simulink model "A14_Servoachse_PID"  (R2017b)
settings: Solver=ode45  StartTime=0.0  StopTime=10  FixedStep=0.001  MaxStep=1e-4  RelTol=1e-3  EnableMultiTasking=on
values from neighbouring files (symbols this model uses):
  CD = 1e1    (= 10)    [A14_Konstanten.m]    (also in A17_Konstanten.m = 100; A8_Konstanten.m = 20; A9_Konstanten.m = 0.1)
  CF = 1e4    (= 10000)    [A13_Konstanten.m]    (also in A14_Konstanten.m; A17_Konstanten.m = 50000; A8_Konstanten.m = 10000000; A9_Konstanten.m)
  CM = 7.1e-7    (= 7.1e-07)    [A10_Konstanten.m]    (also in A13_Konstanten.m; A14_Konstanten.m; A16_Konstanten.m)
  CR = 0.2    [A13_Konstanten.m]    (also in A14_Konstanten.m; A17_Konstanten.m = 100; A9_Konstanten.m = 1; Z_Parametrisierung_Skript.m = [0.5,1,5])
  FReib = 0.5    [A13_Konstanten.m]    (also in A14_Konstanten.m)
  Imax = 4.81    [A10_Konstanten.m]    (also in A13_Konstanten.m; A14_Konstanten.m; A16_Konstanten.m)
  JM = JR + JG    (= 1.38e-06)    [A13_Konstanten.m]    (also in A14_Konstanten.m)
  KM = 38.4e-3    (= 0.0384)    [A10_Konstanten.m]    (also in A13_Konstanten.m; A14_Konstanten.m; A16_Konstanten.m)
  KN = 1/(2*pi*KM)    (= 4.14465997635)    [A10_Konstanten.m]    (also in A13_Konstanten.m; A14_Konstanten.m; A16_Konstanten.m)
  LA = 4.64e-4    (= 0.000464)    [A10_Konstanten.m]    (also in A13_Konstanten.m; A14_Konstanten.m; A16_Konstanten.m)
  m1 = 1    [A13_Konstanten.m]    (also in A14_Konstanten.m; A17_Konstanten.m = 4; A8_Konstanten.m = 20)
  R = 0.02    [A10_Konstanten.m]    (also in A13_Konstanten.m = 0.04; A14_Konstanten.m = 0.04; A16_Konstanten.m)
  RA = 4.99    [A10_Konstanten.m]    (also in A13_Konstanten.m; A14_Konstanten.m; A16_Konstanten.m)
  TPWM = 2e-5    (= 2e-05)    [A14_Konstanten.m]
  Tssens = Tnsens    (= 8e-05)    [A14_Konstanten.m]
  Ue = 4    [A13_Konstanten.m]    (also in A14_Konstanten.m)
  Umax = 24    [A10_Konstanten.m]    (also in A13_Konstanten.m; A14_Konstanten.m; A16_Konstanten.m; A17_Konstanten.m = 120)
  WGrad = 0.85    [A13_Konstanten.m]    (also in A14_Konstanten.m)
undefined symbols (not defined in the file or in its folder): sigbuilder_block
libraries: simulink x2
settings Model: Creator=jbaur  LastModifiedBy=jbaur
settings DataIOCC: ExternalInput=X1  SaveFormat=StructureWithTime  InspectSignalLogs=on  SignalLoggingName=sigsOut
settings OptimizationCC: DefaultParameterBehavior=Inlined  InlineInvariantSignals=on  BufferReuse=off  ExpressionDepthLimit=2147483647  InitFltsAndDblsToZero=on  LifeSpan=inf
settings DebuggingCC: SaveWithParameterizedLinksMsg=none  SignalResolutionControl=TryResolveAllWithWarning  MultiTaskDSMMsg=warning  MultiTaskCondExecSysMsg=none  StateNameClashWarn=warning  InitInArrayFormatMsg=none  SFUnexpectedBacktrackingDiag=warning  SFNoUnconditionalDefaultTransitionDiag=warning  SFExecutionAtInitializationDiag=none
settings HardwareCC: ProdBitPerPointer=32  ProdBitPerSizeT=32  ProdBitPerPtrDiffT=32  ProdLargestAtomicFloat=None  ProdIntDivRoundTo=Undefined  ProdEndianess=Unspecified  ProdWordSize=32  ProdHWDeviceType=32-bit Generic  TargetUnknown=on
settings ModelReferenceCC: PropagateSignalLabelsOutOfModel=off
settings CodeAppCC: StateflowObjectComments=on
settings GRTTargetCC: TargetFcnLib=ansi_tfl_tmw.mat  TargetLangStandard=C89/C90 (ANSI)  ModelReferenceCompliant=off  GeneratePreprocessorConditionals=Disable all  CombineOutputUpdateFcns=off  MatFileLogging=off  GRTInterface=on
settings ConfigComp: CovMetricSettings=dw  CovHtmlReporting=on  CovSaveCumulativeToWorkspaceVar=on  CovSaveSingleToWorkspaceVar=on  CovExternalEMLEnable=off  CovSFcnEnable=off

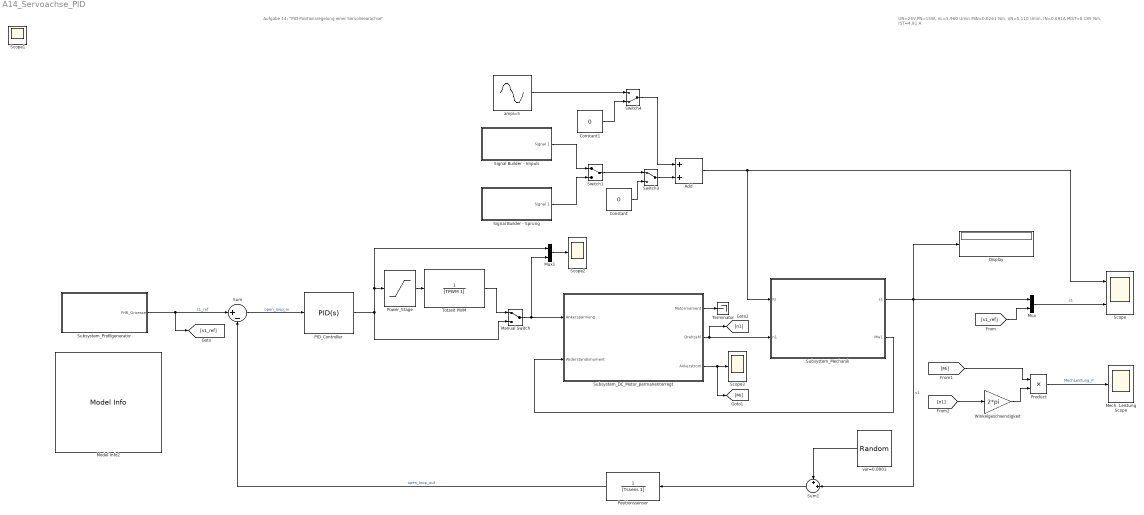
== system A14_Servoachse_PID ==
  note: Aufgabe 14: "PID-Positionsregelung einer Servolinearachse"
  note: UN=24V,PN=15W, nL=5.960 Umin
      | MiN=0.0261 Nm, nN=5.110 Umin, IN=0.691A
      | MiST=0.185 Nm, IST=4.81 A
  Add : Sum
  Constant : Constant  Value=0
  Constant1 : Constant  Value=0
  Display : Display
  Manual Switch : ManualSwitch
  Mech. Leistung Scope : Scope
  Model Info2 : simulink/Model-Wide Utilities/Model Info  Frame=on  DisplayStringWithTags=|  HorizontalTextAlignment=Left  LeftAlignmentValue=0.02
      | Bewegungsprofil:
      | ------------------------
      | Tmax = 1s
      | smax = 0,5m
      | vmax = 1 m/s
      | amax = 2 m/s^2
  Mux : Mux  Inputs=2
  Mux1 : Mux  Inputs=2
  PID_Controller : simulink/Continuous/PID Controller  Controller=PID  TimeDomain=Continuous-time  SampleTime=-1  IntegratorMethod=Forward Euler  FilterMethod=Forward Euler  Form=Ideal  UseFilter=on  ControllerParametersSource=internal  P=10  I=1  D=0  N=1000  InitialConditionSource=internal  InitialConditionForIntegrator=0  InitialConditionForFilter=0  ExternalReset=none  LimitOutput=off  UpperSaturationLimit=Umax  LowerSaturationLimit=-Umax  LinearizeAsGain=off  AntiWindupMode=clamping  Kb=1  TrackingMode=off  Kt=1  PParamMin=[]  PParamMax=[]  IParamMin=[]  IParamMax=[]  DParamMin=[]  DParamMax=[]  NParamMin=[]  NParamMax=[]  KbParamMin=[]  KbParamMax=[]  KtParamMin=[]  KtParamMax=[]  POutMin=[]  POutMax=[]  IOutMin=[]  IOutMax=[]  DOutMin=[]  DOutMax=[]  NOutMin=[]  NOutMax=[]  KbOutMin=[]  KbOutMax=[]  KtOutMin=[]  KtOutMax=[]  IntegratorOutMin=[]  IntegratorOutMax=[]  FilterOutMin=[]  FilterOutMax=[]  SumOutMin=[]  SumOutMax=[]  SumI1OutMin=[]  SumI1OutMax=[]  SumI2OutMin=[]  SumI2OutMax=[]  SumI3OutMin=[]  SumI3OutMax=[]  SumDOutMin=[]  SumDOutMax=[]  SaturationOutMin=[]  SaturationOutMax=[]  IntegratorContinuousStateAttributes=''  IntegratorStateMustResolveToSignalObject=off  IntegratorRTWStateStorageClass=Auto  FilterContinuousStateAttributes=''  FilterStateMustResolveToSignalObject=off  FilterRTWStateStorageClass=Auto  DifferentiatorICPrevScaledInput=0  DifferentiatorOutMin=[]  DifferentiatorOutMax=[]  InitialConditionSetting=State (most efficient)  FilterDiffOutCoefMin=[]  FilterDiffOutCoefMax=[]  SumDenOutMin=[]  SumDenOutMax=[]  SumNumOutMin=[]  SumNumOutMax=[]  ReciprocalOutMin=[]  ReciprocalOutMax=[]  DivideOutMin=[]  DivideOutMax=[]  TunerSelectOption=Transfer Function Based (PID Tuner App)
  Positionssensor : TransferFcn  Denominator=[Tssens 1]
  Power_Stage : Saturate  UpperLimit=Umax  LowerLimit=-Umax
  Product : Product  RndMeth=Zero
  Scope : Scope  NumInputPorts=2
  Scope2 : Scope
  Scope3 : Scope
  Signal Builder - Impuls : Subsystem  Tag=STV Subsys  LoadFcn=sigbuilder_block('load');  StartFcn=sigbuilder_block('start');  StopFcn=sigbuilder_block('stop');  ClipboardFcn=sigbuilder_block('clipboard');  mask(Sigbuilder block){tuvar=[0:10]}
      mask help: Simulink:masks:SigbuilderBlock_MD
      mask init:
      | if ~strcmp(get_param(bdroot(gcbh),'SimulationStatus'),'stopped') tuvar = sigbuilder_block('maskInit'); end
      settings: CopyFcn=sigbuilder_block('copy');  DeleteFcn=sigbuilder_block('delete');  ModelCloseFcn=sigbuilder_block('modelClose');  PreSaveFcn=sigbuilder_block('preSave');  PauseFcn=sigbuilder_block('pause');  ContinueFcn=sigbuilder_block('continue');  NameChangeFcn=sigbuilder_block('namechange');  OpenFcn=sigbuilder_block('open',[431.25 106.5 550.5 399.75 ]);  CloseFcn=sigbuilder_block('close');
      mask Display: plot(0, 0, 100, 100,[2, 2, 32, 32, 2], [68, 8, 8, 68, 68],[32, 2], [38, 38], [32, 19, 2],[53, 60, 44], [32, 17, 17, 2],[16, 16, 31, 31]);txt = getActiveGroup(gcbh);text(2, 100, txt,'verticalAlignment', 'top');
  Signal Builder - Sprung : Subsystem  Tag=STV Subsys  LoadFcn=sigbuilder_block('load');  StartFcn=sigbuilder_block('start');  StopFcn=sigbuilder_block('stop');  ClipboardFcn=sigbuilder_block('clipboard');  mask(Sigbuilder block){tuvar=[0:10]}
      mask help: Simulink:masks:SigbuilderBlock_MD
      mask init:
      | if ~strcmp(get_param(bdroot(gcbh),'SimulationStatus'),'stopped') tuvar = sigbuilder_block('maskInit'); end
      settings: CopyFcn=sigbuilder_block('copy');  DeleteFcn=sigbuilder_block('delete');  ModelCloseFcn=sigbuilder_block('modelClose');  PreSaveFcn=sigbuilder_block('preSave');  PauseFcn=sigbuilder_block('pause');  ContinueFcn=sigbuilder_block('continue');  NameChangeFcn=sigbuilder_block('namechange');  OpenFcn=sigbuilder_block('open',[1699.5 180.75 550.5 399.75 ]);  CloseFcn=sigbuilder_block('close');
      mask Display: plot(0, 0, 100, 100,[2, 2, 32, 32, 2], [68, 8, 8, 68, 68],[32, 2], [38, 38], [32, 19, 2],[53, 60, 44], [32, 17, 17, 2],[16, 16, 31, 31]);txt = getActiveGroup(gcbh);text(2, 100, txt,'verticalAlignment', 'top');
  Subsystem_DC_Motor_permanenterregt : Subsystem
  Subsystem_Mechanik : Subsystem
  Subsystem_Profilgenerator : Subsystem
  Sum : Sum  Inputs=|+-  SaturateOnIntegerOverflow=on
  Sum1 : Sum  Inputs=++|
  Switch1 : ManualSwitch
  Switch3 : ManualSwitch
  Switch4 : ManualSwitch  CurrentSetting=0
  Terminator : Terminator
  Totzeit PWM : TransferFcn  Denominator=[TPWM 1]
  Winkelgeschwindigkeit : Gain  Gain=2*pi
  ampl=5 : Sin  Amplitude=5  Frequency=2*pi*20  SampleTime=0
  var=0.0001 : RandomNumber  Variance=0  SampleTime=0.001
  Scope1 : Scope
  wires:
  Sum/1 -> PID_Controller/1  "open_loop_in"
  Subsystem_Profilgenerator/1(FHR_Groesse) -> Sum/1, [s1_ref]  "s1_ref"
  Mux/1 -> Scope/2  "s1"
  Power_Stage/1 -> Totzeit PWM/1
  Manual Switch/1 -> Subsystem_DC_Motor_permanenterregt/1(Ankerspannung), Mux1/2
  Subsystem_DC_Motor_permanenterregt/2(Drehzahl) -> Subsystem_Mechanik/2(n1), [n1]
  Subsystem_Mechanik/2(Mw1) -> Subsystem_DC_Motor_permanenterregt/2(Widerstandsmoment)
  Mux1/1 -> Scope2/1
  PID_Controller/1 -> Manual Switch/2, Mux1/1, Power_Stage/1
  Subsystem_Mechanik/1(s1) -> Sum1/2, Display/1, Mux/1  "s1"
  Subsystem_DC_Motor_permanenterregt/3(Ankerstrom) -> [Mi], Scope3/1
  [s1_ref] -> Mux/2
  Product/1 -> Mech. Leistung Scope/1  "MechLeistung_P"
  [Mi] -> Product/1
  [n1] -> Winkelgeschwindigkeit/1
  Winkelgeschwindigkeit/1 -> Product/2
  var=0.0001/1 -> Sum1/1
  Sum1/1 -> Positionssensor/1
  Signal Builder - Impuls/1(Signal 1) -> Switch1/1
  Signal Builder - Sprung/1(Signal 1) -> Switch1/2
  Add/1 -> Subsystem_Mechanik/1(Fz), Scope/1
  Switch3/1 -> Add/2
  Switch1/1 -> Switch3/1
  Constant/1 -> Switch3/2
  Switch4/1 -> Add/1
  Constant1/1 -> Switch4/2
  ampl=5/1 -> Switch4/1
  Positionssensor/1 -> Sum/2  "open_loop_out"
  Totzeit PWM/1 -> Manual Switch/1
  Subsystem_DC_Motor_permanenterregt/1(Motormoment) -> Terminator/1

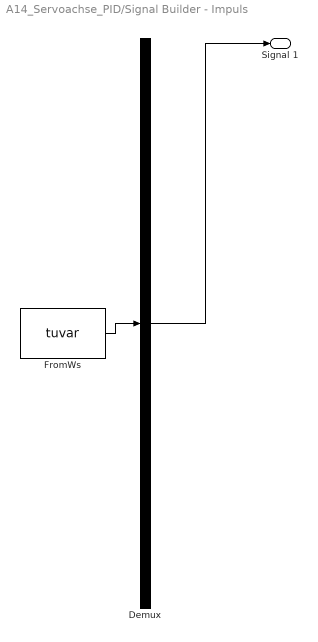
== system A14_Servoachse_PID/Signal Builder - Impuls ==
  Demux : Demux  Tag=STV Demux  Outputs=1
  FromWs : FromWorkspace  Tag=STV FromWs  VariableName=tuvar  SampleTime=0
      SigBuilderData=|
      | common.afterFinalStr = 'Extrapolate'
      | common.sampleTime = 0
      | dataSet.timeRange = [0 20]
      | dataSet.name = 'Group 1'
      | sbobj.Groups.Name = 'Group 1'
      | sbobj.Groups.Signals.Name = 'Signal 1'
      | sbobj.Groups.Signals.XData = [0 5 5 7 7 20]
      | sbobj.Groups.Signals.YData = [0 0 10 10 0 0]
      | sbobj.Groups.TimeRange = [0 20]
  Signal 1 : Outport  Tag=STV Outport
  wires:
  Demux/1 -> Signal 1/1
  FromWs/1 -> Demux/1

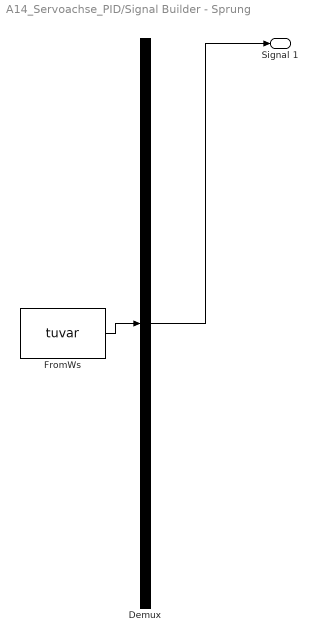
== system A14_Servoachse_PID/Signal Builder - Sprung ==
  Demux : Demux  Tag=STV Demux  Outputs=1
  FromWs : FromWorkspace  Tag=STV FromWs  VariableName=tuvar  SampleTime=0
      SigBuilderData=|
      | common.afterFinalStr = 'Extrapolate'
      | common.sampleTime = 0
      | dataSet.timeRange = [0 20]
      | dataSet.name = 'Group 1'
      | sbobj.Groups.Name = 'Group 1'
      | sbobj.Groups.Signals.Name = 'Signal 1'
      | sbobj.Groups.Signals.XData = [0 5 5 20]
      | sbobj.Groups.Signals.YData = [0 0 10 10]
      | sbobj.Groups.TimeRange = [0 20]
  Signal 1 : Outport  Tag=STV Outport
  wires:
  Demux/1 -> Signal 1/1
  FromWs/1 -> Demux/1

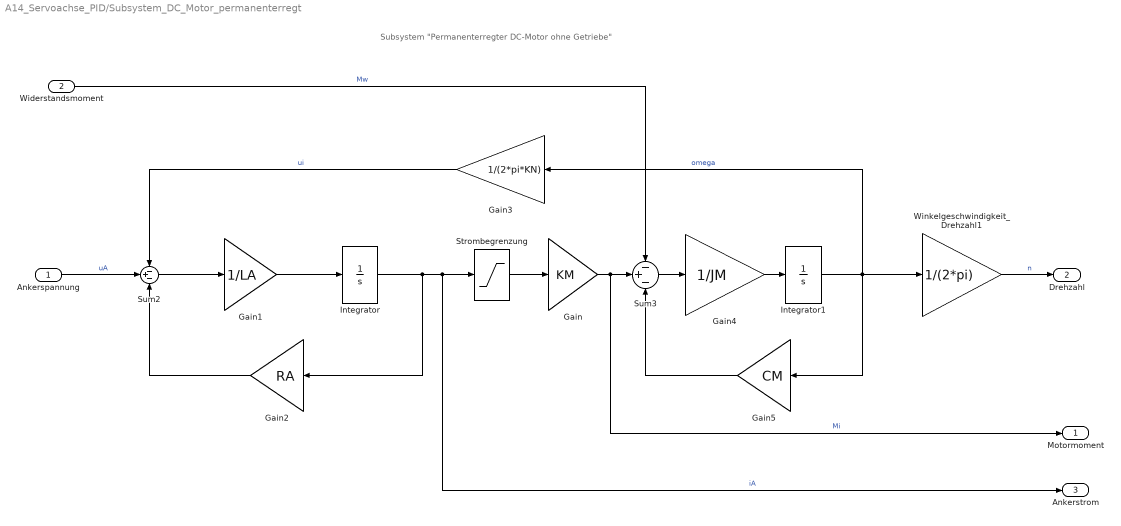
== system A14_Servoachse_PID/Subsystem_DC_Motor_permanenterregt ==
  note: Subsystem "Permanenterregter DC-Motor ohne Getriebe"
  Ankerspannung : Inport
  Widerstandsmoment : Inport  Port=2
  Gain : Gain  Gain=KM
  Gain1 : Gain  Gain=1/LA
  Gain2 : Gain  Gain=RA
  Gain3 : Gain  Gain=1/(2*pi*KN)
  Gain4 : Gain  Gain=1/JM
  Gain5 : Gain  Gain=CM
  Integrator : Integrator
  Integrator1 : Integrator
  Strombegrenzung : Saturate  UpperLimit=Imax  LowerLimit=-Imax
  Sum2 : Sum  Inputs=-+-
  Sum3 : Sum  Inputs=-+-
  Winkelgeschwindigkeit_Drehzahl1 : Gain  Gain=1/(2*pi)
  Motormoment : Outport
  Drehzahl : Outport  Port=2
  Ankerstrom : Outport  Port=3
  wires:
  Ankerspannung/1 -> Sum2/2  "uA"
  Gain3/1 -> Sum2/1  "ui"
  Gain/1 -> Sum3/2, Motormoment/1  "Mi"
  Winkelgeschwindigkeit_Drehzahl1/1 -> Drehzahl/1  "n"
  Sum2/1 -> Gain1/1
  Gain1/1 -> Integrator/1
  Integrator/1 -> Gain2/1, Strombegrenzung/1, Ankerstrom/1  "iA"
  Sum3/1 -> Gain4/1
  Gain4/1 -> Integrator1/1
  Integrator1/1 -> Gain3/1, Winkelgeschwindigkeit_Drehzahl1/1, Gain5/1  "omega"
  Gain5/1 -> Sum3/3
  Gain2/1 -> Sum2/3
  Widerstandsmoment/1 -> Sum3/1  "Mw"
  Strombegrenzung/1 -> Gain/1

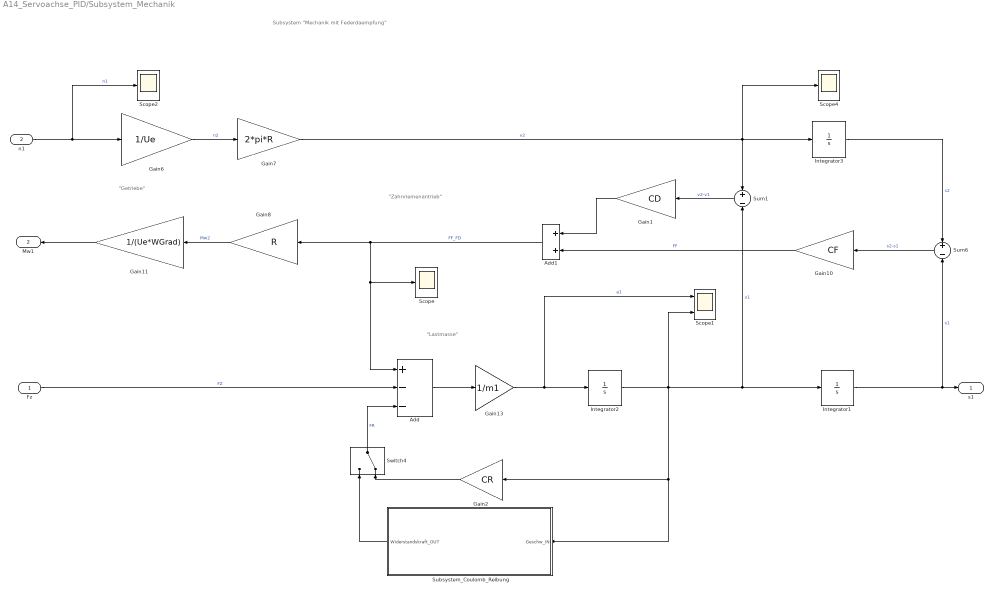
== system A14_Servoachse_PID/Subsystem_Mechanik ==
  note: Subsystem "Mechanik mit Federdaempfung"
  note: "Lastmasse"
  note: "Zahnriemenantrieb"
  note: "Getriebe"
  Fz : Inport
  n1 : Inport  Port=2
  Add : Sum  Inputs=+--
  Add1 : Sum
  Gain1 : Gain  Gain=CD
  Gain10 : Gain  Gain=CF
  Gain11 : Gain  Gain=1/(Ue*WGrad)
  Gain13 : Gain  Gain=1/m1
  Gain2 : Gain  Gain=CR
  Gain6 : Gain  Gain=1/Ue
  Gain7 : Gain  Gain=2*pi*R
  Gain8 : Gain  Gain=R
  Integrator1 : Integrator
  Integrator2 : Integrator
  Integrator3 : Integrator
  Scope : Scope
  Scope1 : Scope  NumInputPorts=2
  Scope2 : Scope
  Scope4 : Scope
  Subsystem_Coulomb_Reibung : Subsystem
  Sum1 : Sum  Inputs=+|-
  Sum6 : Sum  Inputs=+|-
  Switch4 : ManualSwitch  CurrentSetting=0
  s1 : Outport
  Mw1 : Outport  Port=2
  wires:
  Integrator1/1 -> s1/1, Sum6/2  "s1"
  Add/1 -> Gain13/1
  Gain13/1 -> Scope1/1, Integrator2/1  "a1"
  Gain7/1 -> Integrator3/1, Scope4/1, Sum1/1  "v2"
  Gain8/1 -> Gain11/1  "Mw2"
  Sum6/1 -> Gain10/1  "s2-s1"
  n1/1 -> Scope2/1, Gain6/1  "n1"
  Gain6/1 -> Gain7/1  "n2"
  Fz/1 -> Add/2  "FZ"
  Gain11/1 -> Mw1/1
  Sum1/1 -> Gain1/1  "v2-v1"
  Gain10/1 -> Add1/2  "FF"
  Gain1/1 -> Add1/1
  Add1/1 -> Scope/1, Add/1, Gain8/1  "FF_FD"
  Integrator3/1 -> Sum6/1  "s2"
  Integrator2/1 -> Subsystem_Coulomb_Reibung/1(Geschw_IN), Gain2/1, Scope1/2, Sum1/2, Integrator1/1  "v1"
  Switch4/1 -> Add/3  "FR"
  Gain2/1 -> Switch4/2
  Subsystem_Coulomb_Reibung/1(Widerstandskraft_OUT) -> Switch4/1

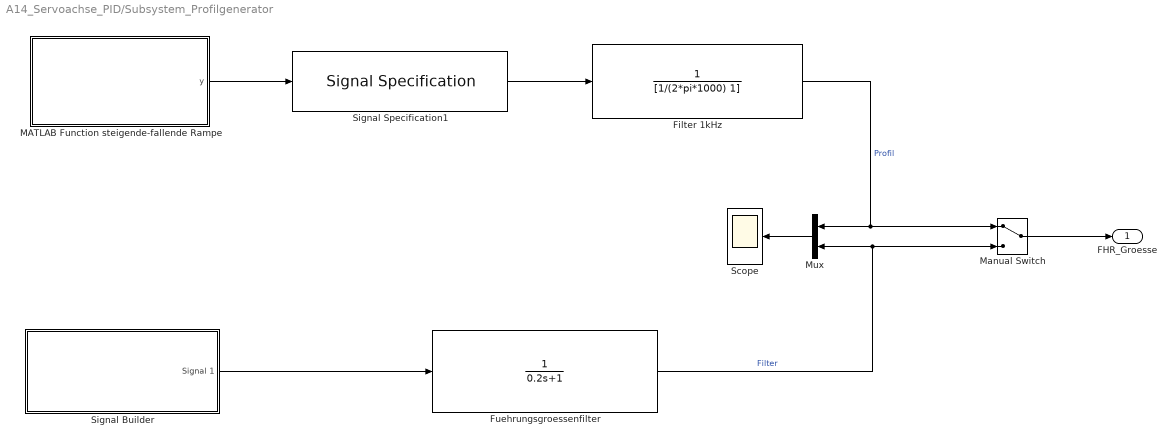
== system A14_Servoachse_PID/Subsystem_Profilgenerator ==
  Filter 1kHz : TransferFcn  Denominator=[1/(2*pi*1000) 1]
  Fuehrungsgroessenfilter : TransferFcn  Denominator=[0.2 1]
  MATLAB Function steigende-fallende Rampe : MATLAB Function  TreatAsAtomicUnit=on
  Manual Switch : ManualSwitch
  Mux : Mux  Inputs=2
  Scope : Scope
  Signal Builder : Subsystem  Tag=STV Subsys  LoadFcn=sigbuilder_block('load');  StartFcn=sigbuilder_block('start');  StopFcn=sigbuilder_block('stop');  ClipboardFcn=sigbuilder_block('clipboard');  mask(Sigbuilder block){tuvar=[0:10]}
      mask help: Simulink:masks:SigbuilderBlock_MD
      mask init:
      | if ~strcmp(get_param(bdroot(gcbh),'SimulationStatus'),'stopped') tuvar = sigbuilder_block('maskInit'); end
      settings: CopyFcn=sigbuilder_block('copy');  DeleteFcn=sigbuilder_block('delete');  ModelCloseFcn=sigbuilder_block('modelClose');  PreSaveFcn=sigbuilder_block('preSave');  PauseFcn=sigbuilder_block('pause');  ContinueFcn=sigbuilder_block('continue');  NameChangeFcn=sigbuilder_block('namechange');  OpenFcn=sigbuilder_block('open',[437.6 199.2 550.4 400 ]);  CloseFcn=sigbuilder_block('close');
      mask Display: plot(0, 0, 100, 100,[2, 2, 32, 32, 2], [68, 8, 8, 68, 68],[32, 2], [38, 38], [32, 19, 2],[53, 60, 44], [32, 17, 17, 2],[16, 16, 31, 31]);txt = getActiveGroup(gcbh);text(2, 100, txt,'verticalAlignment', 'top');
  Signal Specification1 : SignalSpecification  SampleTime=1e-4
  FHR_Groesse : Outport
  wires:
  MATLAB Function steigende-fallende Rampe/1(y) -> Signal Specification1/1
  Signal Specification1/1 -> Filter 1kHz/1
  Manual Switch/1 -> FHR_Groesse/1
  Filter 1kHz/1 -> Mux/1, Manual Switch/1  "Profil"
  Signal Builder/1(Signal 1) -> Fuehrungsgroessenfilter/1
  Fuehrungsgroessenfilter/1 -> Manual Switch/2, Mux/2  "Filter"
  Mux/1 -> Scope/1

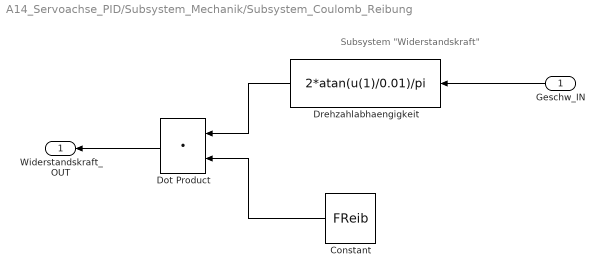
== system A14_Servoachse_PID/Subsystem_Mechanik/Subsystem_Coulomb_Reibung ==
  note: Subsystem "Widerstandskraft"
  Geschw_IN : Inport
  Constant : Constant  Value=FReib
  Dot Product : DotProduct  InputSameDT=on  OutDataTypeStr=Inherit: Inherit via internal rule
  Drehzahlabhaengigkeit : Fcn  Expr=2*atan(u(1)/0.01)/pi
  Widerstandskraft_OUT : Outport
  wires:
  Constant/1 -> Dot Product/2
  Drehzahlabhaengigkeit/1 -> Dot Product/1
  Geschw_IN/1 -> Drehzahlabhaengigkeit/1
  Dot Product/1 -> Widerstandskraft_OUT/1

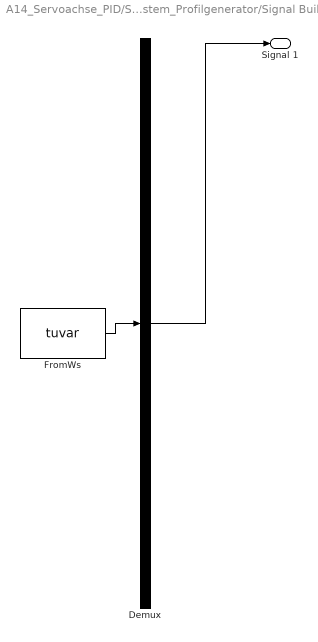
== system A14_Servoachse_PID/Subsystem_Profilgenerator/Signal Builder ==
  Demux : Demux  Tag=STV Demux  Outputs=1
  FromWs : FromWorkspace  Tag=STV FromWs  VariableName=tuvar  SampleTime=0
      SigBuilderData=|
      | common.afterFinalStr = 'Extrapolate'
      | common.sampleTime = 0
      | dataSet.timeRange = [0 10]
      | dataSet.name = 'Group 1'
      | sbobj.Groups.Name = 'Group 1'
      | sbobj.Groups.Signals.Name = 'Signal 1'
      | sbobj.Groups.Signals.XData = [0 1 2 8 8 10]
      | sbobj.Groups.Signals.YData = [0 0 0.5 0.5 0 0]
  Signal 1 : Outport  Tag=STV Outport
  wires:
  Demux/1 -> Signal 1/1
  FromWs/1 -> Demux/1

== matlab function A14_Servoachse_PID/Subsystem_Profilgenerator/MATLAB Function steigende-fallende Rampe ==
  data: y output
function y = Zeitfunktion

% Deklaration der persistenten (globalen) Zeitvariablen
Timestep = 1e-4;
persistent t

% Definition der Zeitfunktion
if isempty(t)
    t=0;
  else
    t = t + Timestep;
end

% Beschleunigungsbegrenztes Bewegungsprofil
T0 = 1;             % Startzeit Vorwärtsfahrt
T1 = 8;             % Startzeit Rückfahrt
s_max = 0.5;
T_max = 1;
t1 = T_max/2;
a_max = s_max/t1^2;
v_max = a_max*t1;

% Bereichsunterscheidung
if t<T0
    y = 0;
else
    if t<=T0+t1
        y = 0.5*a_max*(t-T0)^2;
    else
        if t <= T0+T_max
            y = 0.5*s_max + v_max*(t-t1-T0) - 0.5*a_max*(t-t1-T0)^2;
        else
            if t <= T1
                y = s_max;
            else
                if t <= T1+t1
                    y = s_max - 0.5*a_max*(t-T1)^2;
                else
                    if t <= T1+T_max
                        y = 0.5*s_max - v_max*(t-t1-T1) + 0.5*a_max*(t-t1-T1)^2;
                    else
                        y = 0;
                    end;
                end;
            end;
        end;
    end;
end;
